simulink model "Cooling_Fan"  (R2016b)
settings: Solver=FixedStepDiscrete  StartTime=0.0  StopTime=inf  FixedStep=CoolgFan.tiSimnTiStep_C.Value  RelTol=1e-3  EnableMultiTasking=on
settings Model: Creator=djuenema  LastModifiedBy=djuenema
settings DataIOCC: SaveFormat=StructureWithTime  SaveOutput=off  DSMLogging=off  VisualizeSimOutput=off  SaveTime=off  SignalLoggingName=Results
settings OptimizationCC: BlockReduction=off  ConditionallyExecuteInputs=off  LifeSpan=inf
settings DebuggingCC: AllowSymbolicDim=off  SFUnexpectedBacktrackingDiag=warning  SFNoUnconditionalDefaultTransitionDiag=warning  SFExecutionAtInitializationDiag=none
settings ModelReferenceCC: ModelReferenceNumInstancesAllowed=Single  PropagateSignalLabelsOutOfModel=off
settings GRTTargetCC: TargetLangStandard=C89/C90 (ANSI)
settings ConfigComp: CovMetricSettings=dw  CovHtmlReporting=on  CovSaveCumulativeToWorkspaceVar=on  CovSaveSingleToWorkspaceVar=on  CovExternalEMLEnable=off

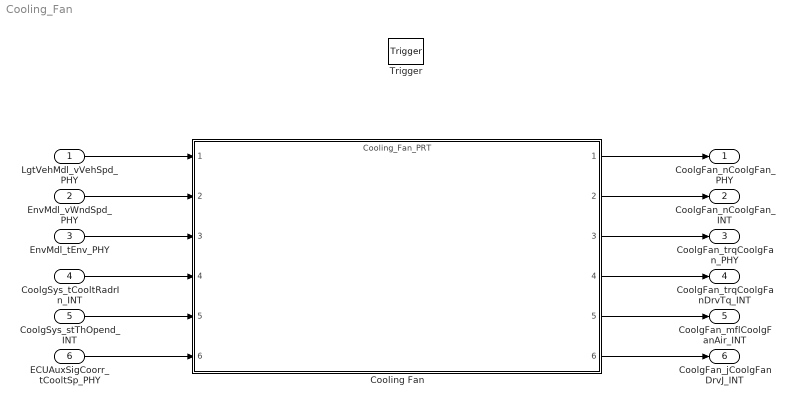
== system Cooling_Fan ==
  LgtVehMdl_vVehSpd_PHY : Inport
  EnvMdl_vWndSpd_PHY : Inport  Port=2
  EnvMdl_tEnv_PHY : Inport  Port=3
  CoolgSys_tCooltRadrIn_INT : Inport  Port=4
  CoolgSys_stThOpend_INT : Inport  Port=5
  ECUAuxSigCoorr_tCooltSp_PHY : Inport  Port=6
  Trigger : TriggerPort  TriggerType=function-call  VariantControl=Variant  PortDimensions=1
  Cooling Fan : ModelReference  ModelNameDialog=Cooling_Fan_PRT.slxp  ModelReferenceVersion=1.3  CopyOfModelProtected=on
  CoolgFan_nCoolgFan_PHY : Outport
  CoolgFan_nCoolgFan_INT : Outport  Port=2
  CoolgFan_trqCoolgFan_PHY : Outport  Port=3
  CoolgFan_trqCoolgFanDrvTq_INT : Outport  Port=4
  CoolgFan_mflCoolgFanAir_INT : Outport  Port=5
  CoolgFan_jCoolgFanDrvJ_INT : Outport  Port=6
  wires:
  EnvMdl_vWndSpd_PHY/1 -> Cooling Fan/2
  LgtVehMdl_vVehSpd_PHY/1 -> Cooling Fan/1
  CoolgSys_stThOpend_INT/1 -> Cooling Fan/5
  CoolgSys_tCooltRadrIn_INT/1 -> Cooling Fan/4
  EnvMdl_tEnv_PHY/1 -> Cooling Fan/3
  Cooling Fan/6 -> CoolgFan_jCoolgFanDrvJ_INT/1
  Cooling Fan/5 -> CoolgFan_mflCoolgFanAir_INT/1
  Cooling Fan/4 -> CoolgFan_trqCoolgFanDrvTq_INT/1
  Cooling Fan/3 -> CoolgFan_trqCoolgFan_PHY/1
  Cooling Fan/2 -> CoolgFan_nCoolgFan_INT/1
  Cooling Fan/1 -> CoolgFan_nCoolgFan_PHY/1
  ECUAuxSigCoorr_tCooltSp_PHY/1 -> Cooling Fan/6
